simulink model "simulink_pid"  (R2014b)
settings: Solver=ode45  StartTime=0.0  StopTime=10  FixedStep=0.1  MaxStep=0.01  RelTol=1e-6
values from neighbouring files (symbols this model uses):
  i_a0 = 0    [main.m]
  J_m = 0.01    [main.m]
  K_E = 1    [main.m]
  K_M = 1    [main.m]
  L_a = 1    [main.m]
  M_L = 0    [main.m]
  R_a = 10    [main.m]
  theta_0 = 0    [main.m]
  theta_r = pi/2    (= 1.57079632679)    [main.m]
  w_m0 = 0    [main.m]
undefined symbols (not defined in the file or in its folder): K_p, T_d, T_i
settings Model: Creator=rende_000  LastModifiedBy=rende_000

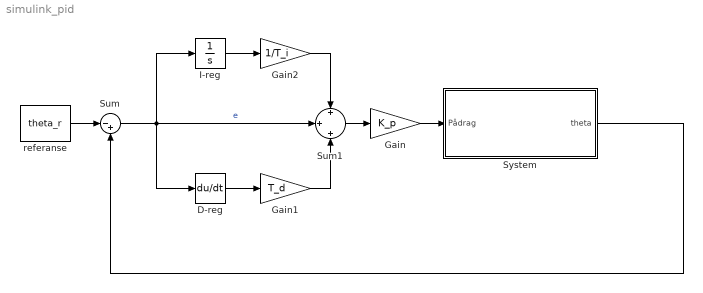
== system simulink_pid ==
  D-reg : Derivative
  Gain : Gain  Gain=K_p
  Gain1 : Gain  Gain=T_d
  Gain2 : Gain  Gain=1/T_i
  I-reg : Integrator
  Sum : Sum  Inputs=|-+
  Sum1 : Sum  Inputs=+|+|+
  System : Subsystem
  referanse : Constant  Value=theta_r
  wires:
  System/1(theta) -> Sum/2
  referanse/1 -> Sum/1
  Sum/1 -> D-reg/1, Sum1/2, I-reg/1  "e"
  D-reg/1 -> Gain1/1
  I-reg/1 -> Gain2/1
  Gain1/1 -> Sum1/3
  Gain2/1 -> Sum1/1
  Sum1/1 -> Gain/1
  Gain/1 -> System/1(Pådrag)

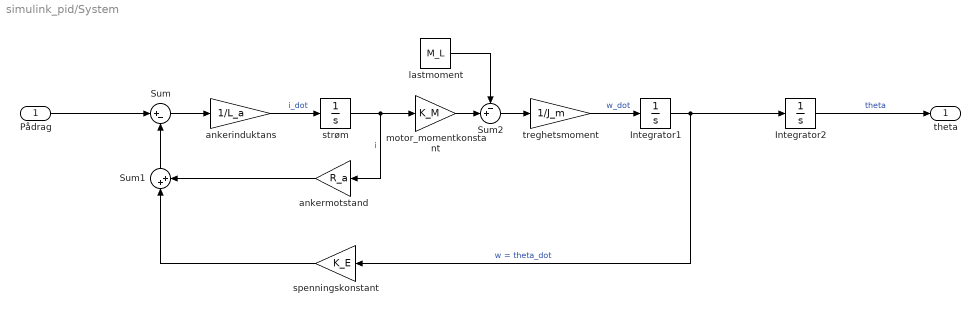
== system simulink_pid/System ==
  Pådrag : Inport
  Integrator1 : Integrator  InitialCondition=w_m0
  Integrator2 : Integrator  InitialCondition=theta_0
  Sum : Sum  Inputs=|+-
  Sum1 : Sum  Inputs=|++
  Sum2 : Sum  Inputs=-+|
  ankerinduktans : Gain  Gain=1/L_a
  ankermotstand : Gain  Gain=R_a
  lastmoment : Constant  Value=M_L
  motor_momentkonstant : Gain  Gain=K_M
  spenningskonstant : Gain  Gain=K_E
  strøm : Integrator  InitialCondition=i_a0
  treghetsmoment : Gain  Gain=1/J_m
  theta : Outport
  wires:
  ankerinduktans/1 -> strøm/1  "i_dot"
  Sum/1 -> ankerinduktans/1
  strøm/1 -> motor_momentkonstant/1, ankermotstand/1  "i"
  Sum2/1 -> treghetsmoment/1
  lastmoment/1 -> Sum2/1
  Integrator1/1 -> spenningskonstant/1, Integrator2/1  "w = theta_dot"
  Sum1/1 -> Sum/2
  ankermotstand/1 -> Sum1/2
  spenningskonstant/1 -> Sum1/1
  Integrator2/1 -> theta/1  "theta"
  motor_momentkonstant/1 -> Sum2/2
  Pådrag/1 -> Sum/1
  treghetsmoment/1 -> Integrator1/1  "w_dot"
